simulink model "SinglePhasInverter"  (R2016a)
settings: Solver=VariableStepAuto  StartTime=0.0  StopTime=1  RelTol=1e-3
libraries: nesl_utility x6, pe_lib x4, fl_lib x3, elec_lib x1
settings Model: Creator=enes_  LastModifiedBy=enes_

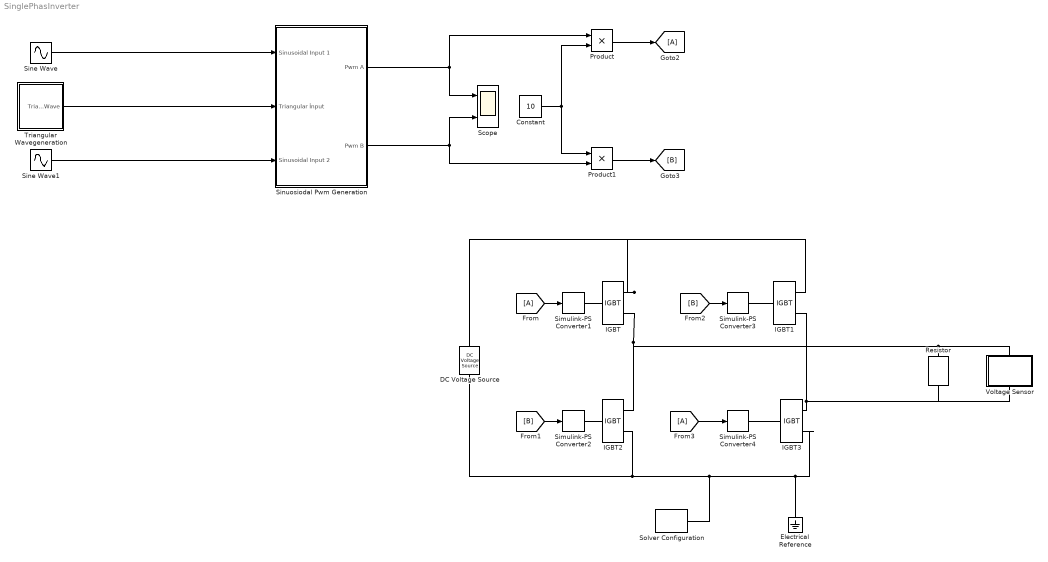
== system SinglePhasInverter ==
  Constant : Constant  Value=10
  DC Voltage Source : fl_lib/Electrical/Electrical Sources/DC Voltage Source  v0=100 V
  Electrical Reference : fl_lib/Electrical/Electrical Elements/Electrical Reference
  IGBT{,1..3} (4 alike) : pe_lib/Semiconductors/Fundamental Components/IGBT  Vf=0.8 V  Ron=0.001 Ohm  Goff=1e-5 1/Ohm  Vth=6 V  diode_param=2  diode_Vf=0.8 V  diode_Ron=0.001 Ohm  diode_Goff=1e-5 1/Ohm  diode_C=5e-8 F  diode_iRM=-235 A  diode_iF=300 A  diode_idot=-50 A/us  diode_trr_param=1  diode_trr_factor=3  diode_trr=15 us  diode_Qrr=1.5e+3 s*uA  thermal_loss_option=2  Voff=300 V  Tau=1e-4 s  Tj=[ 298.15 398.15 ] K  Iout_data=[ 0 10 50 100 200 400 600 ] A  Eon_data=[ 0 2.9e-4 0.00143 0.00286 0.00571 0.01314 0.02286; 0 5.7e-4 0.00263 0.00514 0.01029 0.02057 0.03029 ] J  Eoff_data=[ 0 2.1e-4 0.00107 0.00214 0.00429 0.009859999999999999 0.01714; 0 4.3e-4 0.00197 0.00386 0.00771 0.01543 0.02271 ] J  Von_data=[ 0 1.1 1.3 1.45 1.75 2.25 2.7; 0 1 1.15 1.35 1.7 2.35 3 ] V
  Product : Product
  Product1 : Product
  Resistor : elec_lib/Passive Devices/Resistor  R=100 Ohm  R_tol=5  enable_R_tol=0  tol_distribution=1  nSigma=4  enable_operating_limits=0  operating_limit_action=2  max_working_voltage=100 V  power_rating=1 W  enable_faults=0  fault_action=1  R_faulted=Inf Ohm  enable_temporal_fault=0  t_fault=1 s  enable_behavioral_fault=0  max_permissible_current=1 A  t_fail_on_current=1 s  noise_mode=0  sample_time=0.001 s  repeatability=1  auto_seed=1673915559  user_seed=0  Tdevice=25 degC  alpha=0.00393 1/K  Tmeas=25 degC  thermal_mass=100 J/K  initial_temperature=25 degC  power_derating_T1=70 degC  power_derating_T2=155 degC  operating_temperature_range_vec=[ -50 150 ] degC
  Scope : Scope  NumInputPorts=2
  Simulink-PS Converter{1..4} (4 alike) : nesl_utility/Simulink-PS Converter  PhysicalDomain=network_engine_domain  SubClassName=ps_input  LeftPortType=input  RightPortType=output  PseudoPeriodic=off  Frequencies=[]  NoiseDistribution=none  NoiseParameters=[]  Unit=1  AffineConversion=off  InputFiltering=off  SimscapeFilterOrder=1  InputFilterTimeConstant=0.001  UdotUserProvided=1
  Sine Wave : Sin  Frequency=2*pi*50  SampleTime=0
  Sine Wave1 : Sin  Frequency=2*pi*50  Phase=pi  SampleTime=0
  Sinuosiodal Pwm Generation : Subsystem
  Solver Configuration : nesl_utility/Solver Configuration  PhysicalDomain=network_engine_domain  SubClassName=solver  LeftPortType=input  RightPortType=generic  Accelerate=off  Tones=[]  Harmonics=[]  SimulateNoise=off  Profile=off  UseLocalSampling=off  EnableSwitchedLinearOptims=on  FrequencyDomain=off  UseCCode=off  RelTol=0.001  AbsTol=1e-06  MinStep=1e-09  ToWorkspace=off  RevertToSquareIcSolve=off  NumHomotopyIterations=100  PhasorMode=off  PhasorModeNumHarmonics=1  OverrideAbsTol=off  DoDC=off  ResidualTolerance=1e-09  UseLocalSolver=off  LocalSolverChoice=NE_BACKWARD_EULER_ADVANCER  LocalSolverSampleTime=0.001  DoFixedCost=off  MaxNonlinIter=3  MaxModeIter=2  LinearAlgebra=Sparse  DelaysMemoryBudget=1024  AutomaticFiltering=on  FilteringTimeConstant=0.001
  Triangular Wavegeneration : Subsystem
  "Voltage Sensor " : Subsystem
  wires:
  [A] -> Simulink-PS Converter1/1
  [B] -> Simulink-PS Converter2/1
  [B] -> Simulink-PS Converter3/1
  [A] -> Simulink-PS Converter4/1
  Product/1 -> [A]
  Product1/1 -> [B]
  Constant/1 -> Product/2, Product1/1
  Sinuosiodal Pwm Generation/2(Pwm B) -> Scope/2, Product1/2
  Sinuosiodal Pwm Generation/1(Pwm A) -> Product/1, Scope/1
  Sine Wave/1 -> Sinuosiodal Pwm Generation/1(Sinusoidal Input 1)
  Triangular Wavegeneration/1(Triangular Wave) -> Sinuosiodal Pwm Generation/2(Triangular İnput)
  Sine Wave1/1 -> Sinuosiodal Pwm Generation/3(Sinusoidal Input 2)
  connections:
  IGBT/RConn1 -- DC Voltage Source/LConn1 -- IGBT1/RConn1
  IGBT1/RConn2 -- Resistor/RConn1 -- "Voltage Sensor "/LConn1 -- IGBT3/RConn1
  IGBT3/LConn1 -- Simulink-PS Converter4/RConn1
  Simulink-PS Converter1/RConn1 -- IGBT/LConn1
  Simulink-PS Converter2/RConn1 -- IGBT2/LConn1
  Simulink-PS Converter3/RConn1 -- IGBT1/LConn1
  Electrical Reference/LConn1 -- IGBT3/RConn2 -- Solver Configuration/RConn1 -- DC Voltage Source/RConn1 -- IGBT2/RConn2
  "Voltage Sensor "/RConn1 -- Resistor/LConn1 -- IGBT/RConn2 -- IGBT2/RConn1

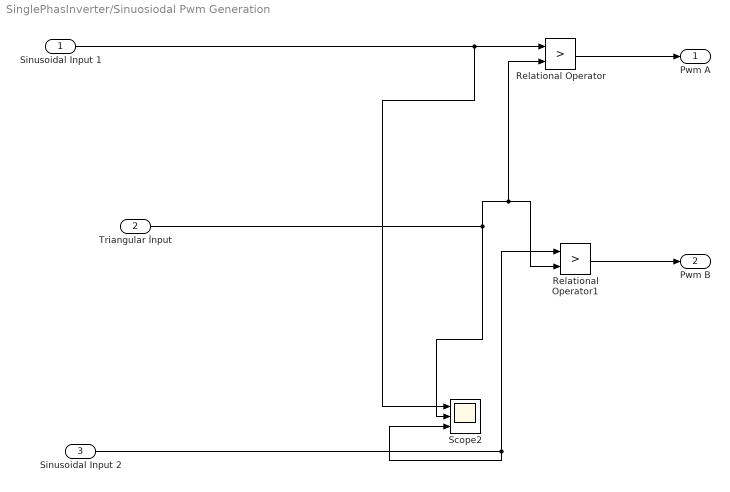
== system SinglePhasInverter/Sinuosiodal Pwm Generation ==
  Sinusoidal Input 1 : Inport
  Triangular İnput : Inport  Port=2
  Sinusoidal Input 2 : Inport  Port=3
  Relational Operator : RelationalOperator  Operator=>  OutDataTypeStr=boolean
  Relational Operator1 : RelationalOperator  Operator=>  OutDataTypeStr=boolean
  Scope2 : Scope  NumInputPorts=3
  Pwm A : Outport
  Pwm B : Outport  Port=2
  wires:
  Sinusoidal Input 2/1 -> Relational Operator1/1, Scope2/3
  Relational Operator/1 -> Pwm A/1
  Sinusoidal Input 1/1 -> Scope2/1, Relational Operator/1
  Relational Operator1/1 -> Pwm B/1
  Triangular İnput/1 -> Relational Operator1/2, Relational Operator/2, Scope2/2

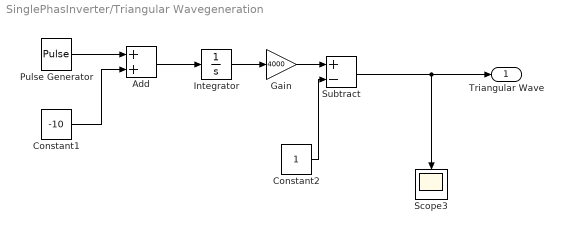
== system SinglePhasInverter/Triangular Wavegeneration ==
  Add : Sum
  Constant1 : Constant  Value=-10
  Constant2 : Constant
  Gain : Gain  Gain=4000
  Integrator : Integrator
  Pulse Generator : DiscretePulseGenerator  PulseType=Time based  Amplitude=20  Period=1/10000  PulseWidth=50
  Scope3 : Scope
  Subtract : Sum  Inputs=+-
  Triangular Wave : Outport
  wires:
  Constant1/1 -> Add/2
  Constant2/1 -> Subtract/2
  Integrator/1 -> Gain/1
  Pulse Generator/1 -> Add/1
  Add/1 -> Integrator/1
  Gain/1 -> Subtract/1
  Subtract/1 -> Triangular Wave/1, Scope3/1

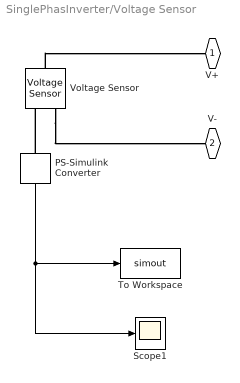
== system SinglePhasInverter/Voltage Sensor  ==
  PS-Simulink Converter : nesl_utility/PS-Simulink Converter  PhysicalDomain=network_engine_domain  SubClassName=ps_output  LeftPortType=input  RightPortType=output  PseudoPeriodic=off  Frequencies=[]  Unit=1  AffineConversion=off
  Scope1 : Scope
  To Workspace : ToWorkspace  VariableName=simout  SaveFormat=Timeseries  SampleTime=-1
  Voltage Sensor : fl_lib/Electrical/Electrical Sensors/Voltage Sensor
  V+ : PMIOPort  Port=1  Side=Right
  V- : PMIOPort  Port=2  Side=Left
  wires:
  PS-Simulink Converter/1 -> Scope1/1, To Workspace/1
  connections:
  PS-Simulink Converter/LConn1 -- Voltage Sensor/RConn1
  Voltage Sensor/RConn2 -- V-/RConn1
  Voltage Sensor/LConn1 -- V+/RConn1
